simulink model "power_PSS_example1"  (R2022a)
settings: Solver=ode23tb  StartTime=0.0  StopTime=25  MaxStep=1/60  RelTol=1e-3  EnableMultiTasking=on
InitFcn:
  | paraset
values from neighbouring files (symbols this model uses):
  delta = 0.1    [paraset.m]
  k = 0.01    [paraset.m]
  kappa = 1    [paraset.m]
undefined symbols (not defined in the file or in its folder): D1, Delta
libraries: spsGenericPowerSystemStabilizerLib x8, spsLoadFlowBusLib x6, spsThreePhaseParallelRLCLoadLib x4, spsThreePhasePISectionLineLib x4, spsSynchronousMachinepuStandardLib x4, spsExcitationSystemLib x4, spsMultiBandPowerSystemStabilizerLib x4, spsSteamTurbineandGovernorLib x4, spsThreePhaseTransformerTwoWindingsLib x4, spsDistributedParametersLineLib x3, spsThreePhaseBreakerLib x2, spsThreePhaseVIMeasurementLib x2
(part 2 of 2)

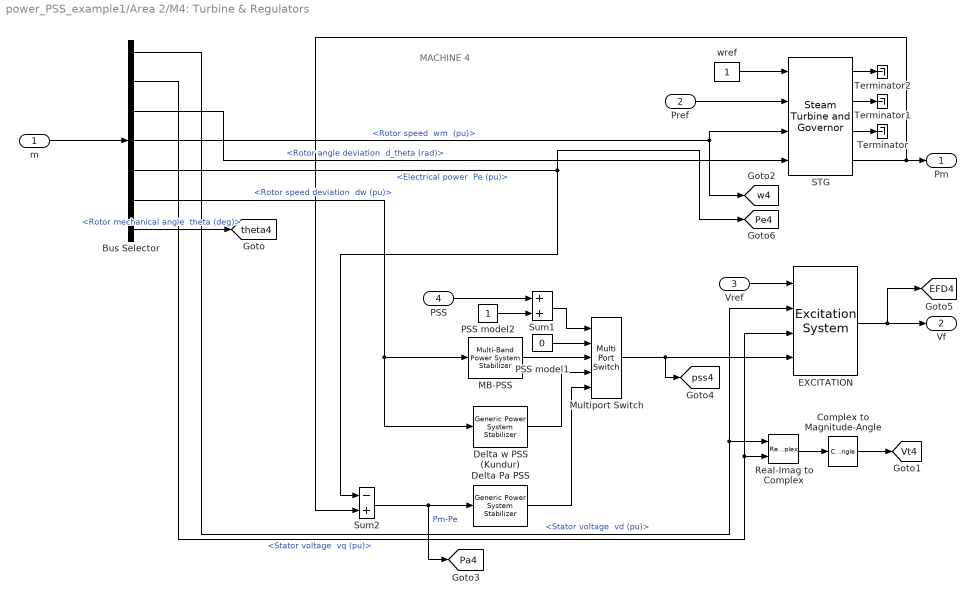
== system power_PSS_example1/Area 2/M4: Turbine & Regulators ==
  note: MACHINE 4
  m : Inport
  Pref : Inport  Port=2
  Vref : Inport  Port=3
  PSS : Inport  Port=4
  Bus Selector : BusSelector  OutputSignals="dq0 components.Stator voltage  vd (pu),dq0 components.Stator voltage  vq (pu),Mechanical.Rotor angle deviation  d_theta (rad),Mechanical.Rotor speed  wm  (pu),Mechanical.Electrical power  Pe (pu),Mechanical.Rotor speed deviation  dw (pu),Mechanical.Rotor mechanical angle  theta (deg)"
  Complex to Magnitude-Angle : ComplexToMagnitudeAngle  Output=Magnitude
  "Delta Pa PSS " : spsGenericPowerSystemStabilizerLib/Generic Power System Stabilizer  Tsensor=15e-3  K=2.5*1.25  Twashout=1  Tleadlag1=[60e-3 1]  Tleadlag2=[0 0]  VSlimits=[-0.15 0.15]  Vinit=0  Plot_On=off  MagdB_On=on  FreqRange=logspace(-2,2,500)
      settings: SourceProductBaseCode=PS
  "Delta w PSS (Kundur) " : spsGenericPowerSystemStabilizerLib/Generic Power System Stabilizer  Tsensor=15e-3  K=30  Twashout=10  Tleadlag1=[50e-3 20e-3]  Tleadlag2=[3 5.4]  VSlimits=[-0.15 0.15]  Vinit=0  Plot_On=off  MagdB_On=on  FreqRange=logspace(-2,2,500)
      settings: SourceProductBaseCode=PS
  EXCITATION : spsExcitationSystemLib/Excitation System  tr=20e-3  reg=[ 200, 0.001 ]  exc=[ 1, 0 ]  tgr=[ 0, 0 ]  damp=[ 0, 0 ]  sat=[ 0, 0 ]  lim=[ 0 , 12.3, 0 ]  v0=[1,1.82209]
      settings: SourceProductBaseCode=PS
  "MB-PSS " : spsMultiBandPowerSystemStabilizerLib/Multi-Band Power System Stabilizer  OperationMode=Simplified settings  Kg=1.0  GL=[0.2 30]  GI=[1.25 40]  GH=[12.0 160]  GLd=[66 66 9.4]  TcLF=[1.667 2 0 0 0 0 2 2.4 0 0 0 0 1 1]  GId=[66 66 47.6]  TcIF=[1 1 0.25 0.3 0 0 1 1 0.3 0.36 0 0 0 0]  GHd=[66 66 233]  TcHF="[0.01 0.012 0 0 0 0  0.012 0.0144 0 0 0 0 1 1]"  LIM=[.075 .15 .15 .15]  Plot_On=off  MagdB_On=off  FreqRange=logspace(-2,2,500)
      settings: SourceProductBaseCode=PS
  Multiport Switch : MultiPortSwitch  Inputs=4  SaturateOnIntegerOverflow=off
  PSS model1 : Constant  Value=0
  PSS model2 : Constant
  Real-Imag to Complex : RealImagToComplex
  STG : spsSteamTurbineandGovernorLib/Steam Turbine and Governor  gentype=Tandem-compound (single mass)  reg1="[ 1  0.05    0 ]"  reg2="[ 0.001  0.15 ]"  reg3="[ -0.1  0.1  0  4.496 ]"  N=3600  turb1="[ 0  10   3.3   0.5   ]"  turb2="[   0   0.36    0.36   0.28   ]"  HA="[ 0.046  1.430  1.465   0.192 ]"  KA="[ 90.44  53.88  64.59   62.94  ]"  DA="[ 0.0115  0.3575  0.3663   0.0137  ]"  ini1=0.7778  ini2=[0.779311,-67.7513]
      settings: SourceProductBaseCode=PS
  Sum1 : Sum  InputSameDT=on  SaturateOnIntegerOverflow=on  OutDataTypeStr=Inherit: Same as first input
  Sum2 : Sum  Inputs=-+  InputSameDT=on  SaturateOnIntegerOverflow=on  OutDataTypeStr=Inherit: Same as first input
  Terminator : Terminator
  Terminator1 : Terminator
  Terminator2 : Terminator
  wref : Constant
  Pm : Outport  InitialOutput=0  VectorParamsAs1DForOutWhenUnconnected=off
  Vf : Outport  Port=2  InitialOutput=0  VectorParamsAs1DForOutWhenUnconnected=off
  tag scope: EFD4=global, Pa4=global, Pe4=global, Vt4=global, pss4=global, theta4=global, w4=global
  wires:
  Bus Selector/1 -> EXCITATION/2, Real-Imag to Complex/1  "<Stator voltage  vd (pu)>"
  Bus Selector/2 -> EXCITATION/3, Real-Imag to Complex/2  "<Stator voltage  vq (pu)>"
  STG/4 -> Pm/1, Sum2/2
  wref/1 -> STG/1
  Pref/1 -> STG/2
  Vref/1 -> EXCITATION/1
  STG/3 -> Terminator/1
  Real-Imag to Complex/1 -> Complex to Magnitude-Angle/1
  EXCITATION/1 -> Vf/1, [EFD4]
  Complex to Magnitude-Angle/1 -> [Vt4]
  Bus Selector/7 -> [theta4]  "<Rotor mechanical angle  theta (deg)>"
  Multiport Switch/1 -> EXCITATION/4, [pss4]
  PSS model1/1 -> Multiport Switch/2
  "MB-PSS "/1 -> Multiport Switch/3
  "Delta w PSS (Kundur) "/1 -> Multiport Switch/4
  "Delta Pa PSS "/1 -> Multiport Switch/5
  PSS model2/1 -> Sum1/2
  Sum1/1 -> Multiport Switch/1
  PSS/1 -> Sum1/1
  Bus Selector/4 -> STG/3, [w4]  "<Rotor speed  wm  (pu)>"
  Bus Selector/5 -> [Pe4], Sum2/1  "<Electrical power  Pe (pu)>"
  Bus Selector/6 -> "MB-PSS "/1, "Delta w PSS (Kundur) "/1  "<Rotor speed deviation  dw (pu)>"
  Sum2/1 -> [Pa4], "Delta Pa PSS "/1  "Pm-Pe"
  STG/2 -> Terminator1/1
  STG/1 -> Terminator2/1
  Bus Selector/3 -> STG/4  "<Rotor angle deviation  d_theta (rad)>"
  m/1 -> Bus Selector/1

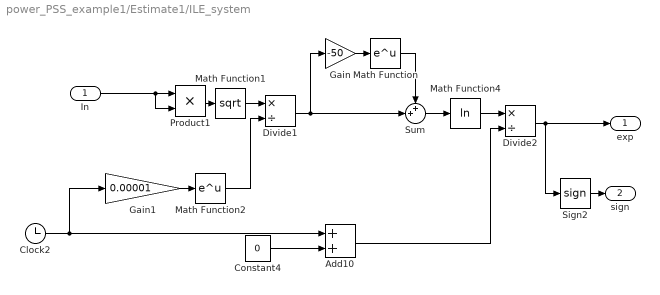
== system power_PSS_example1/Estimate1/ILE_system ==
  In : Inport
  Add10 : Sum
  Clock2 : Clock
  Constant4 : Constant  Value=0
  Divide1 : Product  Inputs=*/
  Divide2 : Product  Inputs=*/
  Gain : Gain  Gain=-50
  Gain1 : Gain  Gain=0.00001
  Math Function : Math  SignedPower=on
  Math Function1 : Math  Operator=sqrt  SignedPower=on
  Math Function2 : Math  SignedPower=on
  Math Function4 : Math  Operator=log  SignedPower=on
  Product1 : Product  RndMeth=Zero
  Sign2 : Signum
  Sum : Sum  Inputs=++|
  exp : Outport  VectorParamsAs1DForOutWhenUnconnected=off
  sign : Outport  Port=2  VectorParamsAs1DForOutWhenUnconnected=off
  wires:
  Gain/1 -> Math Function/1
  Math Function/1 -> Sum/1
  Sum/1 -> Math Function4/1
  Sign2/1 -> sign/1
  Clock2/1 -> Add10/1, Gain1/1
  Divide2/1 -> exp/1, Sign2/1
  Math Function4/1 -> Divide2/1
  Product1/1 -> Math Function1/1
  In/1 -> Product1/1, Product1/2
  Gain1/1 -> Math Function2/1
  Math Function1/1 -> Divide1/1
  Divide1/1 -> Sum/2, Gain/1
  Math Function2/1 -> Divide1/2
  Constant4/1 -> Add10/2
  Add10/1 -> Divide2/2

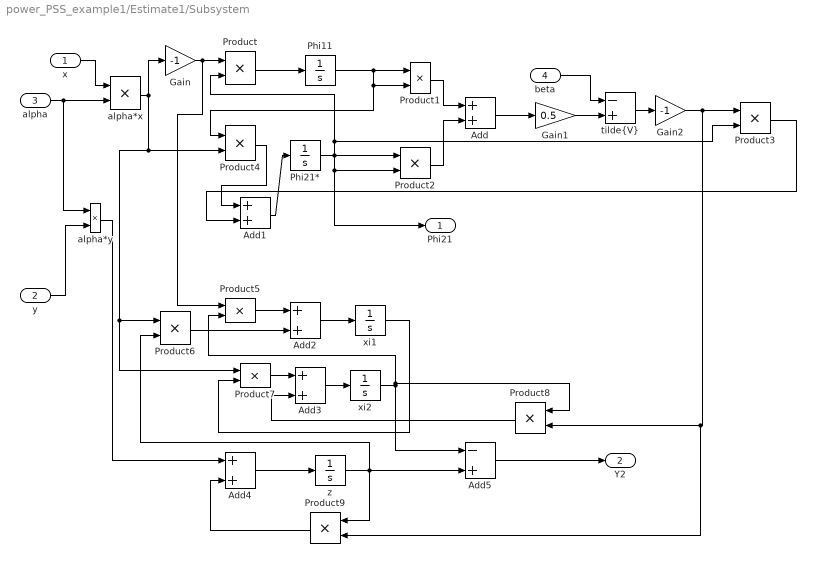
== system power_PSS_example1/Estimate1/Subsystem ==
  x : Inport
  y : Inport  Port=2
  alpha : Inport  Port=3
  beta : Inport  Port=4
  Add{,1..4} (5 alike) : Sum
  Add5 : Sum  Inputs=-+
  Gain : Gain  Gain=-1
  Gain1 : Gain  Gain=0.5
  Gain2 : Gain  Gain=-1
  Phi11 : Integrator  InitialCondition=1
  Phi21* : Integrator
  Product{,1..9} (10 alike) : Product
  alpha*x : Product
  alpha*y : Product
  "tilde{V}" : Sum  Inputs=-+
  xi1 : Integrator
  xi2 : Integrator
  z : Integrator
  Phi21 : Outport
  Y2 : Outport  Port=2
  wires:
  z/1 -> Add5/2, Product9/1, Product6/2
  Product9/1 -> Add4/2
  Phi21*/1 -> Product2/1, Phi21/1, Product2/2, Product/2, Product3/2
  alpha/1 -> alpha*x/2, alpha*y/1
  Gain/1 -> Product/1, Product5/1
  Phi11/1 -> Product1/1, Product4/1, Product1/2
  Add3/1 -> xi2/1
  Product8/1 -> Add3/2
  xi2/1 -> Product8/1, Product5/2, Add5/1
  Gain2/1 -> Product9/2, Product8/2, Product3/1
  Product7/1 -> Add3/1
  Add4/1 -> z/1
  Product/1 -> Phi11/1
  Gain1/1 -> "tilde{V}"/2
  Add1/1 -> Phi21*/1
  Product3/1 -> Add1/2
  Product2/1 -> Add/2
  Product1/1 -> Add/1
  "tilde{V}"/1 -> Gain2/1
  alpha*x/1 -> Product6/1, Product7/1, Product4/2, Gain/1
  Add2/1 -> xi1/1
  Add/1 -> Gain1/1
  xi1/1 -> Product7/2
  Product5/1 -> Add2/1
  beta/1 -> "tilde{V}"/1
  Product4/1 -> Add1/1
  x/1 -> alpha*x/1
  Product6/1 -> Add2/2
  y/1 -> alpha*y/2
  Add5/1 -> Y2/1
  alpha*y/1 -> Add4/1

== system power_PSS_example1/Estimate1/Subsystem1 ==
  signal : Inport
  Add11 : Sum
  Clock2 : Clock
  Constant5 : Constant  Value=5
  Divide2 : Product  Inputs=*/
  Integrator6 : Integrator
  average : Outport
  wires:
  Clock2/1 -> Add11/1
  signal/1 -> Divide2/1
  Divide2/1 -> Integrator6/1
  Integrator6/1 -> average/1
  Constant5/1 -> Add11/2
  Add11/1 -> Divide2/2

== system power_PSS_example1/Estimate1/differential tracker1 ==
  note: hat_x
  note: theta1
  note: Design the gain of kight blue gain blocks!
  signal : Inport
  -gamma1 : Gain  Gain=-1000  SaturateOnIntegerOverflow=on  OutDataTypeStr=Inherit: Same as input  ParamDataTypeStr=Inherit: Same as input
  Integrator1 : Integrator
  Integrator2 : Integrator
  Product2 : Product  SaturateOnIntegerOverflow=on  OutDataTypeStr=Inherit: Same as first input
  Product4 : Product  SaturateOnIntegerOverflow=on  OutDataTypeStr=Inherit: Same as first input
  Sum2 : Sum  Inputs=-+  SaturateOnIntegerOverflow=on
  Sum3 : Sum  SaturateOnIntegerOverflow=on
  e : Scope
  k : Gain  Gain=-55  SaturateOnIntegerOverflow=on  OutDataTypeStr=Inherit: Same as input  ParamDataTypeStr=Inherit: Same as input
  xi : Constant
  diff_estimate : Outport  VectorParamsAs1DForOutWhenUnconnected=off
  wires:
  Integrator2/1 -> -gamma1/1
  Product2/1 -> Integrator2/1
  Sum2/1 -> e/1, k/1, Product2/2
  xi/1 -> Product4/1, Product2/1
  -gamma1/1 -> Product4/2
  k/1 -> Sum3/2
  Product4/1 -> Sum3/1, diff_estimate/1
  Integrator1/1 -> Sum2/2
  Sum3/1 -> Integrator1/1
  signal/1 -> Sum2/1

== system power_PSS_example1/Estimate1/differential tracker2 ==
  note: hat_x
  note: theta1
  note: Design the gain of kight blue gain blocks!
  signal : Inport
  -gamma1 : Gain  Gain=-1000  SaturateOnIntegerOverflow=on  OutDataTypeStr=Inherit: Same as input  ParamDataTypeStr=Inherit: Same as input
  Integrator1 : Integrator
  Integrator2 : Integrator
  Product2 : Product  SaturateOnIntegerOverflow=on  OutDataTypeStr=Inherit: Same as first input
  Product4 : Product  SaturateOnIntegerOverflow=on  OutDataTypeStr=Inherit: Same as first input
  Sum2 : Sum  Inputs=-+  SaturateOnIntegerOverflow=on
  Sum3 : Sum  SaturateOnIntegerOverflow=on
  e : Scope
  k : Gain  Gain=-55  SaturateOnIntegerOverflow=on  OutDataTypeStr=Inherit: Same as input  ParamDataTypeStr=Inherit: Same as input
  xi : Constant
  diff_estimate : Outport  VectorParamsAs1DForOutWhenUnconnected=off
  wires:
  Integrator2/1 -> -gamma1/1
  Product2/1 -> Integrator2/1
  Sum2/1 -> e/1, k/1, Product2/2
  xi/1 -> Product4/1, Product2/1
  -gamma1/1 -> Product4/2
  k/1 -> Sum3/2
  Product4/1 -> Sum3/1, diff_estimate/1
  Integrator1/1 -> Sum2/2
  Sum3/1 -> Integrator1/1
  signal/1 -> Sum2/1

== matlab function power_PSS_example1/Estimate1/MATLAB Function ==
  data: u input; y output
function y = fcn(u)
  delta = 0.5;
y = abs(u)^delta*sign(u);
